simulink model "motors"  (R2020b)
settings: Solver=VariableStepAuto  StartTime=0.0  StopTime=10.0  RelTol=1e-3
libraries: fl_lib x33, nesl_utility x14, ee_lib x13
settings Model: Creator=jbmic  LastModifiedBy=jbmic

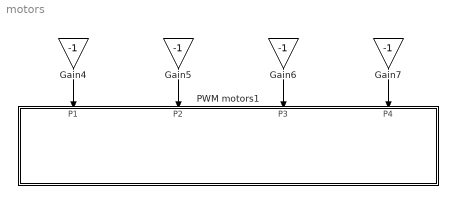
== system motors ==
  Gain{4..7} (4 alike) : Gain  Gain=-1
  PWM motors1 : Subsystem
  wires:
  Gain7/1 -> PWM motors1/4(P4)
  Gain5/1 -> PWM motors1/2(P2)
  Gain4/1 -> PWM motors1/1(P1)
  Gain6/1 -> PWM motors1/3(P3)

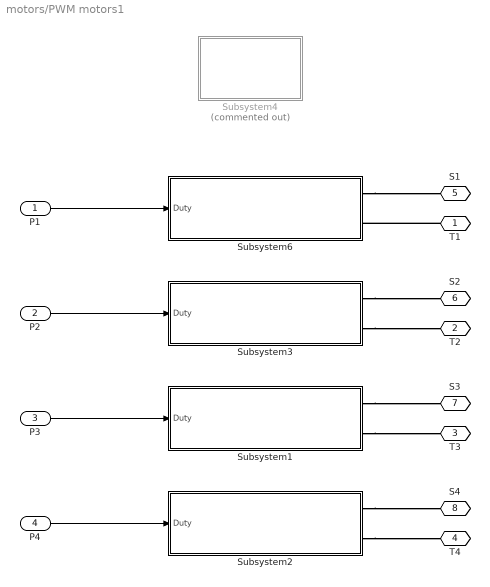
== system motors/PWM motors1 ==
  P1 : Inport
  P2 : Inport  Port=2
  P3 : Inport  Port=3
  P4 : Inport  Port=4
  Subsystem1 : Subsystem
  Subsystem2 : Subsystem
  Subsystem3 : Subsystem
  Subsystem4 : Subsystem  Commented=on
  Subsystem6 : Subsystem
  T1 : PMIOPort  Side=Right
  T2 : PMIOPort  Port=2  Side=Right
  T3 : PMIOPort  Port=3  Side=Right
  T4 : PMIOPort  Port=4  Side=Right
  S1 : PMIOPort  Port=5  Side=Right
  S2 : PMIOPort  Port=6  Side=Right
  S3 : PMIOPort  Port=7  Side=Right
  S4 : PMIOPort  Port=8  Side=Right
  wires:
  P1/1 -> Subsystem6/1(Duty)
  P2/1 -> Subsystem3/1(Duty)
  P3/1 -> Subsystem1/1(Duty)
  P4/1 -> Subsystem2/1(Duty)
  connections:
  Subsystem2/RConn2 -- T4/RConn1
  Subsystem6/RConn1 -- S1/RConn1
  Subsystem1/RConn2 -- T3/RConn1
  Subsystem1/RConn1 -- S3/RConn1
  T1/RConn1 -- Subsystem6/RConn2
  Subsystem3/RConn1 -- S2/RConn1
  Subsystem3/RConn2 -- T2/RConn1
  Subsystem2/RConn1 -- S4/RConn1

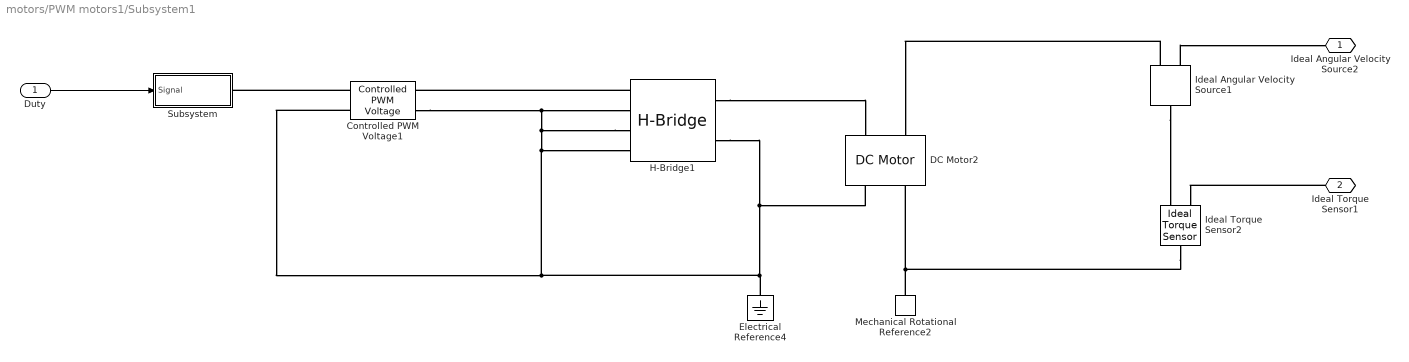
== system motors/PWM motors1/Subsystem1 ==
  Duty : Inport
  Controlled PWM Voltage1 : ee_lib/Integrated Circuits/Controlled PWM Voltage  F=1000 Hz  TD=0 s  pulse_width_offset=0 s  pulse_min=0 s  Vmin=0 V  Vmax=12 V  Vm=5 V  pwm_or_av=2  event_type=1  sample_time=1e-6 s  u_min=0  u_max=1
  DC Motor2 : ee_lib/Electromechanical/Brushed Motors/DC Motor  field_option=ee.enum.field_option.pm  Rf=100 Ohm  Lf=1 H  Laf=0.15 H  If0=0 A  parameterization=ee.enum.dcparam_option.torque_speed  Ra=13 Ohm  La=0.6 mH  emf_or_torque=ee.enum.emf_or_torque.kv  Kv=0.0098 V/(rad/s)  Ki=6.876e-4 N*m/A  T_stall=0.00988 N*m  w_max=11090 rpm  w_rated=15000 rpm  P_rated=0.08 W  V_rated=12 V  J=0.106 g*cm^2  lam_param=ee.enum.lam_param.damping  lam=1e-6 N*m/(rad/s)  i_noload=0 A  V_i_noload=1.5 V  speed0=0 rpm  enable_fault_armature=ee.enum.faults.faultEnable.no  rev_faulted=1 / 3  G_faulted_armature=1e-5 S  fault_trigger_armature=ee.enum.faults.faultTrigger.temporal  t_fault_armature=1 s  max_permissible_current_armature=inf A  t_fail_on_current_armature=1 s  enable_fault_field=ee.enum.faults.faultEnable.no  G_faulted_field=1e-5 S  fault_trigger_field=ee.enum.faults.faultTrigger.temporal  t_fault_field=1 s  max_permissible_current_field=inf A  t_fail_on_current_field=1 s  fault_action=ee.enum.faults.faultAction.none  alpha=3.93e-3 1/K  Tmeas=25 degC  thermal_mass=100 J/K  initial_temperature=25 degC
  Electrical Reference4 : fl_lib/Electrical/Electrical Elements/Electrical Reference
  H-Bridge1 : ee_lib/Semiconductors & Converters/Converters/H-Bridge  supply_ports=ee.enum.supply_ports.hidesupply  Venable=2.5 V  Vmax=5.0 V  Vreverse=2.5 V  Vbrake=2.5 V  Vm=12 V  pwm_or_av=ee.enum.pwm_or_av.averaged  regenerative_braking_mode=ee.enum.converters.regenerative_braking_mode.always_enabled  discontinuous=ee.enum.current_profile.continuous  freewheeling_mode=ee.enum.converters.freewheeling_mode.one_switch_one_diode  Ron=0.1 Ohm  Don=0.1 Ohm  Goff=1e-6 S  Rload=10 Ohm  Lload=1e-5 H  F=10 kHz  thermal_mass=100 J/K  initial_temperature=298.15 K  Ron2=0.1 Ohm  Don2=0.05 Ohm  Tmeas=298.15 K  Tmeas2=398.15 K
  Ideal Angular Velocity Source1 : fl_lib/Mechanical/Mechanical Sources/Ideal Angular Velocity Source
  Ideal Torque Sensor2 : fl_lib/Mechanical/Mechanical Sensors/Ideal Torque Sensor
  Mechanical Rotational Reference2 : fl_lib/Mechanical/Rotational Elements/Mechanical Rotational Reference
  Subsystem : Subsystem
  Ideal Angular Velocity Source2 : PMIOPort  Side=Right
  Ideal Torque Sensor1 : PMIOPort  Port=2  Side=Right
  wires:
  Duty/1 -> Subsystem/1(Signal)
  connections:
  H-Bridge1/RConn1 -- DC Motor2/LConn1
  Ideal Torque Sensor2/LConn1 -- DC Motor2/RConn2 -- Mechanical Rotational Reference2/LConn1
  H-Bridge1/LConn3 -- Controlled PWM Voltage1/RConn2 -- H-Bridge1/LConn2 -- H-Bridge1/LConn4 -- Controlled PWM Voltage1/LConn2 -- Electrical Reference4/LConn1 -- H-Bridge1/RConn2 -- DC Motor2/RConn1
  Ideal Torque Sensor1/RConn1 -- Ideal Torque Sensor2/RConn2
  H-Bridge1/LConn1 -- Controlled PWM Voltage1/RConn1
  Controlled PWM Voltage1/LConn1 -- Subsystem/RConn1
  Ideal Angular Velocity Source1/LConn1 -- Ideal Torque Sensor2/RConn1
  Ideal Angular Velocity Source1/RConn2 -- DC Motor2/LConn2
  Ideal Angular Velocity Source1/RConn1 -- Ideal Angular Velocity Source2/RConn1

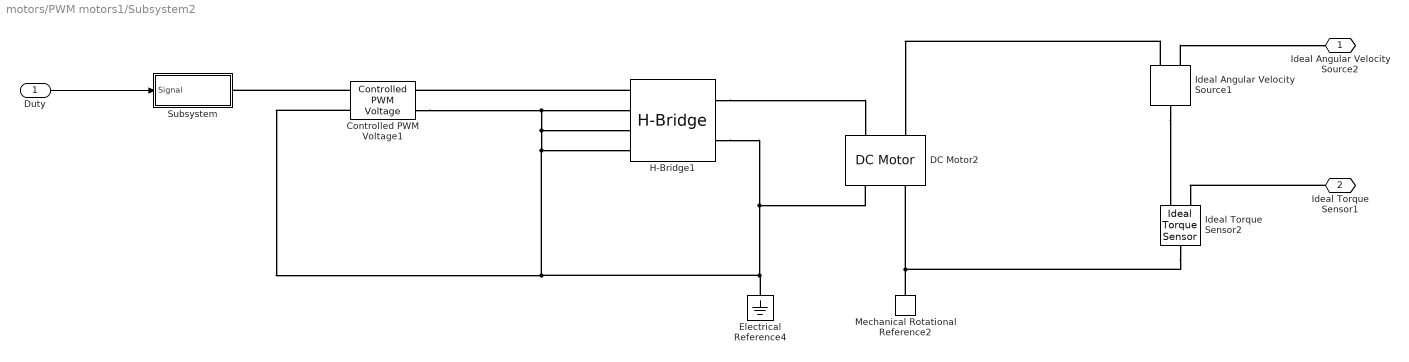
== system motors/PWM motors1/Subsystem2 ==
  Duty : Inport
  Controlled PWM Voltage1 : ee_lib/Integrated Circuits/Controlled PWM Voltage  F=1000 Hz  TD=0 s  pulse_width_offset=0 s  pulse_min=0 s  Vmin=0 V  Vmax=12 V  Vm=5 V  pwm_or_av=2  event_type=1  sample_time=1e-6 s  u_min=0  u_max=1
  DC Motor2 : ee_lib/Electromechanical/Brushed Motors/DC Motor  field_option=ee.enum.field_option.pm  Rf=100 Ohm  Lf=1 H  Laf=0.15 H  If0=0 A  parameterization=ee.enum.dcparam_option.torque_speed  Ra=13 Ohm  La=0.6 mH  emf_or_torque=ee.enum.emf_or_torque.kv  Kv=0.0098 V/(rad/s)  Ki=6.876e-4 N*m/A  T_stall=0.00988 N*m  w_max=11090 rpm  w_rated=15000 rpm  P_rated=0.08 W  V_rated=12 V  J=0.106 g*cm^2  lam_param=ee.enum.lam_param.damping  lam=1e-6 N*m/(rad/s)  i_noload=0 A  V_i_noload=1.5 V  speed0=0 rpm  enable_fault_armature=ee.enum.faults.faultEnable.no  rev_faulted=1 / 3  G_faulted_armature=1e-5 S  fault_trigger_armature=ee.enum.faults.faultTrigger.temporal  t_fault_armature=1 s  max_permissible_current_armature=inf A  t_fail_on_current_armature=1 s  enable_fault_field=ee.enum.faults.faultEnable.no  G_faulted_field=1e-5 S  fault_trigger_field=ee.enum.faults.faultTrigger.temporal  t_fault_field=1 s  max_permissible_current_field=inf A  t_fail_on_current_field=1 s  fault_action=ee.enum.faults.faultAction.none  alpha=3.93e-3 1/K  Tmeas=25 degC  thermal_mass=100 J/K  initial_temperature=25 degC
  Electrical Reference4 : fl_lib/Electrical/Electrical Elements/Electrical Reference
  H-Bridge1 : ee_lib/Semiconductors & Converters/Converters/H-Bridge  supply_ports=ee.enum.supply_ports.hidesupply  Venable=2.5 V  Vmax=5.0 V  Vreverse=2.5 V  Vbrake=2.5 V  Vm=12 V  pwm_or_av=ee.enum.pwm_or_av.averaged  regenerative_braking_mode=ee.enum.converters.regenerative_braking_mode.always_enabled  discontinuous=ee.enum.current_profile.continuous  freewheeling_mode=ee.enum.converters.freewheeling_mode.one_switch_one_diode  Ron=0.1 Ohm  Don=0.1 Ohm  Goff=1e-6 S  Rload=10 Ohm  Lload=1e-5 H  F=10 kHz  thermal_mass=100 J/K  initial_temperature=298.15 K  Ron2=0.1 Ohm  Don2=0.05 Ohm  Tmeas=298.15 K  Tmeas2=398.15 K
  Ideal Angular Velocity Source1 : fl_lib/Mechanical/Mechanical Sources/Ideal Angular Velocity Source
  Ideal Torque Sensor2 : fl_lib/Mechanical/Mechanical Sensors/Ideal Torque Sensor
  Mechanical Rotational Reference2 : fl_lib/Mechanical/Rotational Elements/Mechanical Rotational Reference
  Subsystem : Subsystem
  Ideal Angular Velocity Source2 : PMIOPort  Side=Right
  Ideal Torque Sensor1 : PMIOPort  Port=2  Side=Right
  wires:
  Duty/1 -> Subsystem/1(Signal)
  connections:
  Ideal Angular Velocity Source1/RConn1 -- Ideal Angular Velocity Source2/RConn1
  Ideal Angular Velocity Source1/RConn2 -- DC Motor2/LConn2
  Ideal Angular Velocity Source1/LConn1 -- Ideal Torque Sensor2/RConn1
  Controlled PWM Voltage1/LConn1 -- Subsystem/RConn1
  H-Bridge1/LConn1 -- Controlled PWM Voltage1/RConn1
  Ideal Torque Sensor1/RConn1 -- Ideal Torque Sensor2/RConn2
  DC Motor2/RConn1 -- H-Bridge1/RConn2 -- Electrical Reference4/LConn1 -- Controlled PWM Voltage1/LConn2 -- H-Bridge1/LConn4 -- H-Bridge1/LConn2 -- Controlled PWM Voltage1/RConn2 -- H-Bridge1/LConn3
  Mechanical Rotational Reference2/LConn1 -- DC Motor2/RConn2 -- Ideal Torque Sensor2/LConn1
  H-Bridge1/RConn1 -- DC Motor2/LConn1

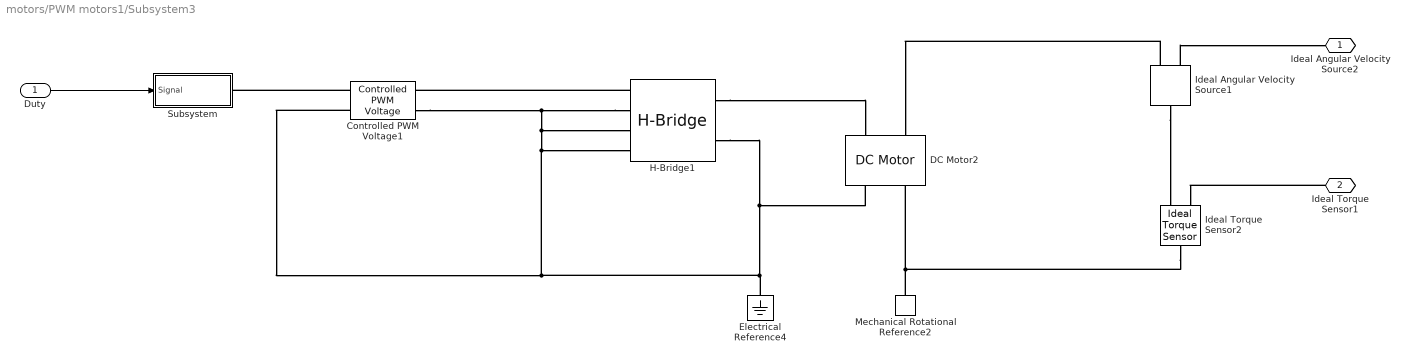
== system motors/PWM motors1/Subsystem3 ==
  Duty : Inport
  Controlled PWM Voltage1 : ee_lib/Integrated Circuits/Controlled PWM Voltage  F=1000 Hz  TD=0 s  pulse_width_offset=0 s  pulse_min=0 s  Vmin=0 V  Vmax=12 V  Vm=5 V  pwm_or_av=2  event_type=1  sample_time=1e-6 s  u_min=0  u_max=1
  DC Motor2 : ee_lib/Electromechanical/Brushed Motors/DC Motor  field_option=ee.enum.field_option.pm  Rf=100 Ohm  Lf=1 H  Laf=0.15 H  If0=0 A  parameterization=ee.enum.dcparam_option.torque_speed  Ra=13 Ohm  La=0.6 mH  emf_or_torque=ee.enum.emf_or_torque.kv  Kv=0.0098 V/(rad/s)  Ki=6.876e-4 N*m/A  T_stall=0.00988 N*m  w_max=11090 rpm  w_rated=15000 rpm  P_rated=0.08 W  V_rated=12 V  J=0.106 g*cm^2  lam_param=ee.enum.lam_param.damping  lam=1e-6 N*m/(rad/s)  i_noload=0 A  V_i_noload=1.5 V  speed0=0 rpm  enable_fault_armature=ee.enum.faults.faultEnable.no  rev_faulted=1 / 3  G_faulted_armature=1e-5 S  fault_trigger_armature=ee.enum.faults.faultTrigger.temporal  t_fault_armature=1 s  max_permissible_current_armature=inf A  t_fail_on_current_armature=1 s  enable_fault_field=ee.enum.faults.faultEnable.no  G_faulted_field=1e-5 S  fault_trigger_field=ee.enum.faults.faultTrigger.temporal  t_fault_field=1 s  max_permissible_current_field=inf A  t_fail_on_current_field=1 s  fault_action=ee.enum.faults.faultAction.none  alpha=3.93e-3 1/K  Tmeas=25 degC  thermal_mass=100 J/K  initial_temperature=25 degC
  Electrical Reference4 : fl_lib/Electrical/Electrical Elements/Electrical Reference
  H-Bridge1 : ee_lib/Semiconductors & Converters/Converters/H-Bridge  supply_ports=ee.enum.supply_ports.hidesupply  Venable=2.5 V  Vmax=5.0 V  Vreverse=2.5 V  Vbrake=2.5 V  Vm=12 V  pwm_or_av=ee.enum.pwm_or_av.averaged  regenerative_braking_mode=ee.enum.converters.regenerative_braking_mode.always_enabled  discontinuous=ee.enum.current_profile.continuous  freewheeling_mode=ee.enum.converters.freewheeling_mode.one_switch_one_diode  Ron=0.1 Ohm  Don=0.1 Ohm  Goff=1e-6 S  Rload=10 Ohm  Lload=1e-5 H  F=10 kHz  thermal_mass=100 J/K  initial_temperature=298.15 K  Ron2=0.1 Ohm  Don2=0.05 Ohm  Tmeas=298.15 K  Tmeas2=398.15 K
  Ideal Angular Velocity Source1 : fl_lib/Mechanical/Mechanical Sources/Ideal Angular Velocity Source
  Ideal Torque Sensor2 : fl_lib/Mechanical/Mechanical Sensors/Ideal Torque Sensor
  Mechanical Rotational Reference2 : fl_lib/Mechanical/Rotational Elements/Mechanical Rotational Reference
  Subsystem : Subsystem
  Ideal Angular Velocity Source2 : PMIOPort  Side=Right
  Ideal Torque Sensor1 : PMIOPort  Port=2  Side=Right
  wires:
  Duty/1 -> Subsystem/1(Signal)
  connections:
  Ideal Angular Velocity Source1/RConn1 -- Ideal Angular Velocity Source2/RConn1
  Ideal Angular Velocity Source1/RConn2 -- DC Motor2/LConn2
  Ideal Angular Velocity Source1/LConn1 -- Ideal Torque Sensor2/RConn1
  Controlled PWM Voltage1/LConn1 -- Subsystem/RConn1
  H-Bridge1/LConn1 -- Controlled PWM Voltage1/RConn1
  Ideal Torque Sensor1/RConn1 -- Ideal Torque Sensor2/RConn2
  H-Bridge1/LConn2 -- H-Bridge1/LConn3 -- DC Motor2/RConn1 -- H-Bridge1/RConn2 -- Electrical Reference4/LConn1 -- Controlled PWM Voltage1/LConn2 -- H-Bridge1/LConn4 -- Controlled PWM Voltage1/RConn2
  Mechanical Rotational Reference2/LConn1 -- DC Motor2/RConn2 -- Ideal Torque Sensor2/LConn1
  H-Bridge1/RConn1 -- DC Motor2/LConn1

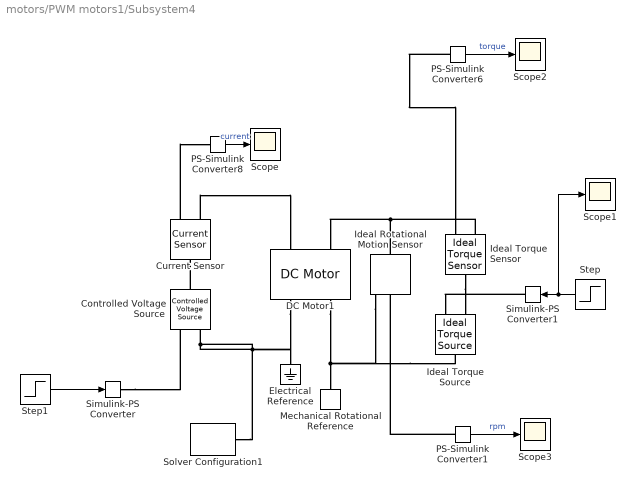
== system motors/PWM motors1/Subsystem4 ==
  Controlled Voltage Source : fl_lib/Electrical/Electrical Sources/Controlled Voltage Source
  Current Sensor : fl_lib/Electrical/Electrical Sensors/Current Sensor
  DC Motor1 : ee_lib/Electromechanical/Brushed Motors/DC Motor  field_option=ee.enum.field_option.pm  Rf=100 Ohm  Lf=1 H  Laf=0.15 H  If0=0 A  parameterization=ee.enum.dcparam_option.torque_speed  Ra=13 Ohm  La=0.6 mH  emf_or_torque=ee.enum.emf_or_torque.kv  Kv=0.0098 V/(rad/s)  Ki=6.876e-4 N*m/A  T_stall=0.00988 N*m  w_max=11090 rpm  w_rated=15000 rpm  P_rated=0.08 W  V_rated=12 V  J=0.106 g*cm^2  lam_param=ee.enum.lam_param.damping  lam=0 N*m/(rad/s)  i_noload=0 A  V_i_noload=1.5 V  speed0=0 rpm  enable_fault_armature=ee.enum.faults.faultEnable.no  rev_faulted=1 / 3  G_faulted_armature=1e-5 S  fault_trigger_armature=ee.enum.faults.faultTrigger.temporal  t_fault_armature=1 s  max_permissible_current_armature=inf A  t_fail_on_current_armature=1 s  enable_fault_field=ee.enum.faults.faultEnable.no  G_faulted_field=1e-5 S  fault_trigger_field=ee.enum.faults.faultTrigger.temporal  t_fault_field=1 s  max_permissible_current_field=inf A  t_fail_on_current_field=1 s  fault_action=ee.enum.faults.faultAction.none  alpha=3.93e-3 1/K  Tmeas=25 degC  thermal_mass=100 J/K  initial_temperature=25 degC
  Electrical Reference : fl_lib/Electrical/Electrical Elements/Electrical Reference
  Ideal Rotational Motion Sensor : fl_lib/Mechanical/Mechanical Sensors/Ideal Rotational Motion Sensor  wrap_angle=simscape.enum.onoff.off  offset=0 rad
  Ideal Torque Sensor : fl_lib/Mechanical/Mechanical Sensors/Ideal Torque Sensor
  Ideal Torque Source : fl_lib/Mechanical/Mechanical Sources/Ideal Torque Source
  Mechanical Rotational Reference : fl_lib/Mechanical/Rotational Elements/Mechanical Rotational Reference
  PS-Simulink Converter1 : nesl_utility/PS-Simulink Converter  PhysicalDomain=network_engine_domain  SubClassName=ps_output  LeftPortType=input  RightPortType=output  PseudoPeriodic=off  Frequencies=[]  Unit=rpm  AffineConversion=off
  PS-Simulink Converter6 : nesl_utility/PS-Simulink Converter  PhysicalDomain=network_engine_domain  SubClassName=ps_output  LeftPortType=input  RightPortType=output  PseudoPeriodic=off  Frequencies=[]  Unit=N*m  AffineConversion=off
  PS-Simulink Converter8 : nesl_utility/PS-Simulink Converter  PhysicalDomain=network_engine_domain  SubClassName=ps_output  LeftPortType=input  RightPortType=output  PseudoPeriodic=off  Frequencies=[]  Unit=A  AffineConversion=off
  Scope{,1..3} (4 alike) : Scope
  Simulink-PS Converter : nesl_utility/Simulink-PS Converter  PhysicalDomain=network_engine_domain  SubClassName=ps_input  LeftPortType=input  RightPortType=output  PseudoPeriodic=off  Frequencies=[]  NoiseDistribution=none  NoiseParameters=[]  Unit=V  AffineConversion=off  FilteringAndDerivatives=provide  SimscapeFilterOrder=1  InputFilterTimeConstant=0.001  UdotUserProvided=0
  Simulink-PS Converter1 : nesl_utility/Simulink-PS Converter  PhysicalDomain=network_engine_domain  SubClassName=ps_input  LeftPortType=input  RightPortType=output  PseudoPeriodic=off  Frequencies=[]  NoiseDistribution=none  NoiseParameters=[]  Unit=N*m  AffineConversion=off  FilteringAndDerivatives=provide  SimscapeFilterOrder=1  InputFilterTimeConstant=0.001  UdotUserProvided=0
  Solver Configuration1 : nesl_utility/Solver Configuration  PhysicalDomain=network_engine_domain  SubClassName=solver  LeftPortType=input  RightPortType=generic  Tones=[]  Harmonics=[]  SimulateNoise=off  Profile=off  UseLocalSampling=off  EnableSwitchedLinearOptims=on  FrequencyDomain=off  UseCCode=off  RelTol=0.001  AbsTol=1e-06  MinStep=1e-09  ToWorkspace=off  RevertToSquareIcSolve=off  NumHomotopyIterations=100  PhasorMode=off  PhasorModeNumHarmonics=1  DoDC=off  ResidualTolerance=1e-09  UseLocalSolver=off  LocalSolverChoice=NE_BACKWARD_EULER_ADVANCER  LocalSolverSampleTime=0.001  DoFixedCost=off  MaxNonlinIter=3  MaxModeIter=2  ComputeImpulses=off  ImpulseIterations=2  LinearAlgebra=auto  EquationFormulation=NE_TIME_EF  DelaysMemoryBudget=1024  AutomaticFiltering=on  FilteringTimeConstant=0.001  PartitionStorageMethod=AS_NEEDED  PartitionMemoryBudget=1024  PartitionMethod=ROBUST
  Step : Step  After=-0.00988  SampleTime=0
  Step1 : Step  Time=0  After=12  SampleTime=0
  wires:
  Step1/1 -> Simulink-PS Converter/1
  PS-Simulink Converter8/1 -> Scope/1  "current"
  Step/1 -> Scope1/1, Simulink-PS Converter1/1
  PS-Simulink Converter6/1 -> Scope2/1  "torque"
  PS-Simulink Converter1/1 -> Scope3/1  "rpm"
  connections:
  Current Sensor/RConn2 -- DC Motor1/LConn1
  Current Sensor/RConn1 -- PS-Simulink Converter8/LConn1
  Ideal Rotational Motion Sensor/LConn1 -- DC Motor1/LConn2 -- Ideal Torque Sensor/RConn1
  PS-Simulink Converter6/LConn1 -- Ideal Torque Sensor/RConn2
  Simulink-PS Converter/RConn1 -- Controlled Voltage Source/RConn1
  Controlled Voltage Source/LConn1 -- Current Sensor/LConn1
  DC Motor1/RConn2 -- Ideal Rotational Motion Sensor/RConn1 -- Ideal Torque Source/LConn1 -- Mechanical Rotational Reference/LConn1
  Controlled Voltage Source/RConn2 -- Electrical Reference/LConn1 -- DC Motor1/RConn1 -- Solver Configuration1/RConn1
  Ideal Torque Sensor/LConn1 -- Ideal Torque Source/RConn2
  Simulink-PS Converter1/RConn1 -- Ideal Torque Source/RConn1
  PS-Simulink Converter1/LConn1 -- Ideal Rotational Motion Sensor/RConn2

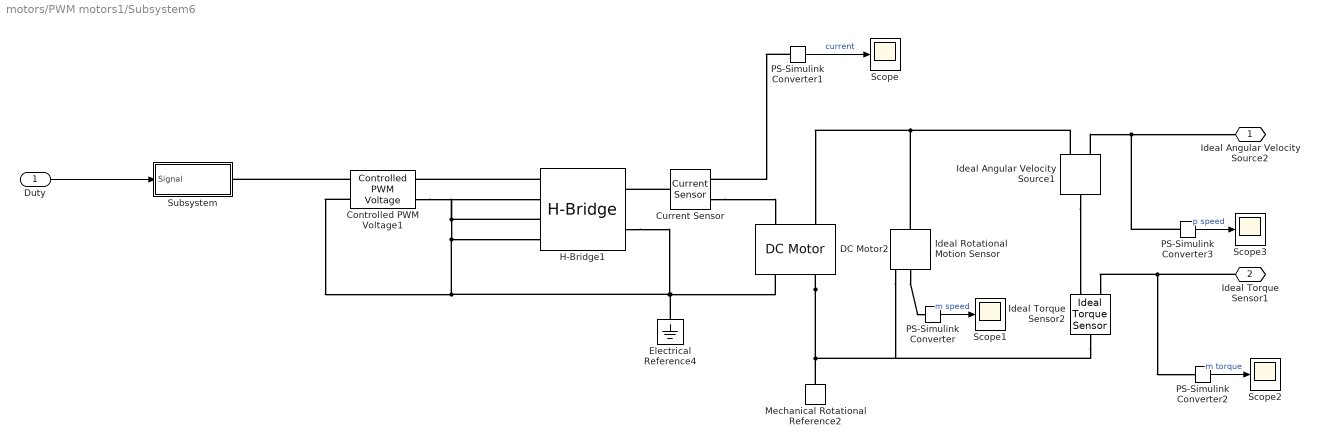
== system motors/PWM motors1/Subsystem6 ==
  Duty : Inport
  Controlled PWM Voltage1 : ee_lib/Integrated Circuits/Controlled PWM Voltage  F=1000 Hz  TD=0 s  pulse_width_offset=0 s  pulse_min=0 s  Vmin=0 V  Vmax=7.4 V  Vm=7.4 V  pwm_or_av=2  event_type=1  sample_time=1e-6 s  u_min=0  u_max=1
  Current Sensor : fl_lib/Electrical/Electrical Sensors/Current Sensor
  DC Motor2 : ee_lib/Electromechanical/Brushed Motors/DC Motor  field_option=ee.enum.field_option.pm  Rf=100 Ohm  Lf=1 H  Laf=0.15 H  If0=0 A  parameterization=ee.enum.dcparam_option.torque_speed  Ra=13 Ohm  La=0.6 mH  emf_or_torque=ee.enum.emf_or_torque.kv  Kv=0.0098 V/(rad/s)  Ki=6.876e-4 N*m/A  T_stall=0.00988 N*m  w_max=11090 rpm  w_rated=15000 rpm  P_rated=0.08 W  V_rated=12 V  J=0.106 g*cm^2  lam_param=ee.enum.lam_param.damping  lam=1e-6 N*m/(rad/s)  i_noload=0 A  V_i_noload=1.5 V  speed0=0 rpm  enable_fault_armature=ee.enum.faults.faultEnable.no  rev_faulted=1 / 3  G_faulted_armature=1e-5 S  fault_trigger_armature=ee.enum.faults.faultTrigger.temporal  t_fault_armature=1 s  max_permissible_current_armature=inf A  t_fail_on_current_armature=1 s  enable_fault_field=ee.enum.faults.faultEnable.no  G_faulted_field=1e-5 S  fault_trigger_field=ee.enum.faults.faultTrigger.temporal  t_fault_field=1 s  max_permissible_current_field=inf A  t_fail_on_current_field=1 s  fault_action=ee.enum.faults.faultAction.none  alpha=3.93e-3 1/K  Tmeas=25 degC  thermal_mass=100 J/K  initial_temperature=25 degC
  Electrical Reference4 : fl_lib/Electrical/Electrical Elements/Electrical Reference
  H-Bridge1 : ee_lib/Semiconductors & Converters/Converters/H-Bridge  supply_ports=ee.enum.supply_ports.hidesupply  Venable=3.7 V  Vmax=7.4 V  Vreverse=3.7 V  Vbrake=3.7 V  Vm=7.4 V  pwm_or_av=ee.enum.pwm_or_av.averaged  regenerative_braking_mode=ee.enum.converters.regenerative_braking_mode.always_enabled  discontinuous=ee.enum.current_profile.continuous  freewheeling_mode=ee.enum.converters.freewheeling_mode.one_switch_one_diode  Ron=0.1 Ohm  Don=0.1 Ohm  Goff=1e-6 S  Rload=10 Ohm  Lload=1e-5 H  F=10 kHz  thermal_mass=100 J/K  initial_temperature=298.15 K  Ron2=0.1 Ohm  Don2=0.05 Ohm  Tmeas=298.15 K  Tmeas2=398.15 K
  Ideal Angular Velocity Source1 : fl_lib/Mechanical/Mechanical Sources/Ideal Angular Velocity Source
  Ideal Rotational Motion Sensor : fl_lib/Mechanical/Mechanical Sensors/Ideal Rotational Motion Sensor  wrap_angle=simscape.enum.onoff.off  offset=0 rad
  Ideal Torque Sensor2 : fl_lib/Mechanical/Mechanical Sensors/Ideal Torque Sensor
  Mechanical Rotational Reference2 : fl_lib/Mechanical/Rotational Elements/Mechanical Rotational Reference
  PS-Simulink Converter : nesl_utility/PS-Simulink Converter  PhysicalDomain=network_engine_domain  SubClassName=ps_output  LeftPortType=input  RightPortType=output  PseudoPeriodic=off  Frequencies=[]  Unit=rpm  AffineConversion=off
  PS-Simulink Converter1 : nesl_utility/PS-Simulink Converter  PhysicalDomain=network_engine_domain  SubClassName=ps_output  LeftPortType=input  RightPortType=output  PseudoPeriodic=off  Frequencies=[]  Unit=inherit  AffineConversion=off
  PS-Simulink Converter2 : nesl_utility/PS-Simulink Converter  PhysicalDomain=network_engine_domain  SubClassName=ps_output  LeftPortType=input  RightPortType=output  PseudoPeriodic=off  Frequencies=[]  Unit=inherit  AffineConversion=off
  PS-Simulink Converter3 : nesl_utility/PS-Simulink Converter  PhysicalDomain=network_engine_domain  SubClassName=ps_output  LeftPortType=input  RightPortType=output  PseudoPeriodic=off  Frequencies=[]  Unit=rpm  AffineConversion=off
  Scope{,1..3} (4 alike) : Scope
  Subsystem : Subsystem
  Ideal Angular Velocity Source2 : PMIOPort  Side=Right
  Ideal Torque Sensor1 : PMIOPort  Port=2  Side=Right
  wires:
  Duty/1 -> Subsystem/1(Signal)
  PS-Simulink Converter1/1 -> Scope/1  "current"
  PS-Simulink Converter/1 -> Scope1/1  "m speed"
  PS-Simulink Converter2/1 -> Scope2/1  "m torque"
  PS-Simulink Converter3/1 -> Scope3/1  "p speed"
  connections:
  Current Sensor/RConn2 -- DC Motor2/LConn1
  DC Motor2/RConn2 -- Ideal Torque Sensor2/LConn1 -- Ideal Rotational Motion Sensor/RConn1 -- Mechanical Rotational Reference2/LConn1
  Electrical Reference4/LConn1 -- Controlled PWM Voltage1/LConn2 -- H-Bridge1/LConn3 -- H-Bridge1/LConn2 -- Controlled PWM Voltage1/RConn2 -- H-Bridge1/LConn4 -- H-Bridge1/RConn2 -- DC Motor2/RConn1
  H-Bridge1/LConn1 -- Controlled PWM Voltage1/RConn1
  Controlled PWM Voltage1/LConn1 -- Subsystem/RConn1
  Ideal Angular Velocity Source1/LConn1 -- Ideal Torque Sensor2/RConn1
  Ideal Angular Velocity Source1/RConn2 -- Ideal Rotational Motion Sensor/LConn1 -- DC Motor2/LConn2
  Current Sensor/LConn1 -- H-Bridge1/RConn1
  PS-Simulink Converter1/LConn1 -- Current Sensor/RConn1
  Ideal Rotational Motion Sensor/RConn2 -- PS-Simulink Converter/LConn1
  Ideal Torque Sensor1/RConn1 -- PS-Simulink Converter2/LConn1 -- Ideal Torque Sensor2/RConn2
  Ideal Angular Velocity Source1/RConn1 -- PS-Simulink Converter3/LConn1 -- Ideal Angular Velocity Source2/RConn1

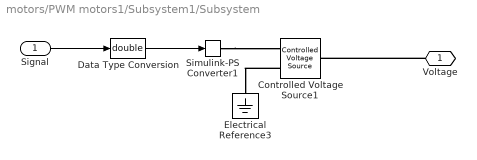
== system motors/PWM motors1/Subsystem1/Subsystem ==
  Signal : Inport
  Controlled Voltage Source1 : fl_lib/Electrical/Electrical Sources/Controlled Voltage Source
  Data Type Conversion : DataTypeConversion  OutDataTypeStr=double
  Electrical Reference3 : fl_lib/Electrical/Electrical Elements/Electrical Reference
  Simulink-PS Converter1 : nesl_utility/Simulink-PS Converter  PhysicalDomain=network_engine_domain  SubClassName=ps_input  LeftPortType=input  RightPortType=output  PseudoPeriodic=off  Frequencies=[]  NoiseDistribution=none  NoiseParameters=[]  Unit=V  AffineConversion=off  FilteringAndDerivatives=zero  SimscapeFilterOrder=1  InputFilterTimeConstant=0.001  UdotUserProvided=0
  Voltage : PMIOPort  Side=Right
  wires:
  Data Type Conversion/1 -> Simulink-PS Converter1/1
  Signal/1 -> Data Type Conversion/1
  connections:
  Controlled Voltage Source1/RConn2 -- Electrical Reference3/LConn1
  Simulink-PS Converter1/RConn1 -- Controlled Voltage Source1/RConn1
  Voltage/RConn1 -- Controlled Voltage Source1/LConn1

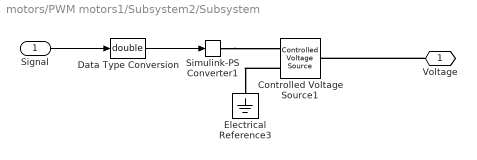
== system motors/PWM motors1/Subsystem2/Subsystem ==
  Signal : Inport
  Controlled Voltage Source1 : fl_lib/Electrical/Electrical Sources/Controlled Voltage Source
  Data Type Conversion : DataTypeConversion  OutDataTypeStr=double
  Electrical Reference3 : fl_lib/Electrical/Electrical Elements/Electrical Reference
  Simulink-PS Converter1 : nesl_utility/Simulink-PS Converter  PhysicalDomain=network_engine_domain  SubClassName=ps_input  LeftPortType=input  RightPortType=output  PseudoPeriodic=off  Frequencies=[]  NoiseDistribution=none  NoiseParameters=[]  Unit=V  AffineConversion=off  FilteringAndDerivatives=zero  SimscapeFilterOrder=1  InputFilterTimeConstant=0.001  UdotUserProvided=0
  Voltage : PMIOPort  Side=Right
  wires:
  Signal/1 -> Data Type Conversion/1
  Data Type Conversion/1 -> Simulink-PS Converter1/1
  connections:
  Voltage/RConn1 -- Controlled Voltage Source1/LConn1
  Simulink-PS Converter1/RConn1 -- Controlled Voltage Source1/RConn1
  Controlled Voltage Source1/RConn2 -- Electrical Reference3/LConn1

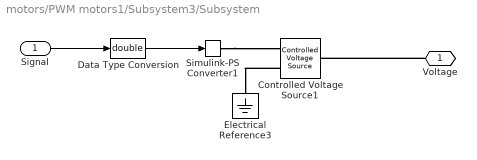
== system motors/PWM motors1/Subsystem3/Subsystem ==
  Signal : Inport
  Controlled Voltage Source1 : fl_lib/Electrical/Electrical Sources/Controlled Voltage Source
  Data Type Conversion : DataTypeConversion  OutDataTypeStr=double
  Electrical Reference3 : fl_lib/Electrical/Electrical Elements/Electrical Reference
  Simulink-PS Converter1 : nesl_utility/Simulink-PS Converter  PhysicalDomain=network_engine_domain  SubClassName=ps_input  LeftPortType=input  RightPortType=output  PseudoPeriodic=off  Frequencies=[]  NoiseDistribution=none  NoiseParameters=[]  Unit=V  AffineConversion=off  FilteringAndDerivatives=zero  SimscapeFilterOrder=1  InputFilterTimeConstant=0.001  UdotUserProvided=0
  Voltage : PMIOPort  Side=Right
  wires:
  Signal/1 -> Data Type Conversion/1
  Data Type Conversion/1 -> Simulink-PS Converter1/1
  connections:
  Voltage/RConn1 -- Controlled Voltage Source1/LConn1
  Simulink-PS Converter1/RConn1 -- Controlled Voltage Source1/RConn1
  Controlled Voltage Source1/RConn2 -- Electrical Reference3/LConn1

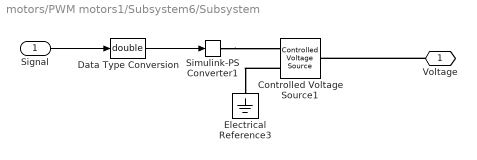
== system motors/PWM motors1/Subsystem6/Subsystem ==
  Signal : Inport
  Controlled Voltage Source1 : fl_lib/Electrical/Electrical Sources/Controlled Voltage Source
  Data Type Conversion : DataTypeConversion  OutDataTypeStr=double
  Electrical Reference3 : fl_lib/Electrical/Electrical Elements/Electrical Reference
  Simulink-PS Converter1 : nesl_utility/Simulink-PS Converter  PhysicalDomain=network_engine_domain  SubClassName=ps_input  LeftPortType=input  RightPortType=output  PseudoPeriodic=off  Frequencies=[]  NoiseDistribution=none  NoiseParameters=[]  Unit=V  AffineConversion=off  FilteringAndDerivatives=zero  SimscapeFilterOrder=1  InputFilterTimeConstant=0.001  UdotUserProvided=0
  Voltage : PMIOPort  Side=Right
  wires:
  Data Type Conversion/1 -> Simulink-PS Converter1/1
  Signal/1 -> Data Type Conversion/1
  connections:
  Controlled Voltage Source1/RConn2 -- Electrical Reference3/LConn1
  Simulink-PS Converter1/RConn1 -- Controlled Voltage Source1/RConn1
  Voltage/RConn1 -- Controlled Voltage Source1/LConn1
